simulink model "OuterController"  (R2016b)
settings: Solver=FixedStepAuto  StartTime=0.0  StopTime=t  FixedStep=0.05  RelTol=1e-3
model workspace (MAT data in the model file):
  index = Simulink.Signal
  index.DataType = 'double'
  index.Dimensions = 1
  index.DimensionsMode = 'Fixed'
  index.Complexity = 'real'
  index.SampleTime = -1
  index.SamplingMode = 'auto'
  index.InitialValue = '1'
values from neighbouring files (symbols this model uses):
  AcceptRadius = 1    [Parameters.m]
  wps = [1 0 ... (first row only)    [Parameters.m]
  xbdot = 0.5    [PlannerResults.m]
settings Model: Creator=USUARIO  LastModifiedBy=USUARIO
settings DataIOCC: Refine=100

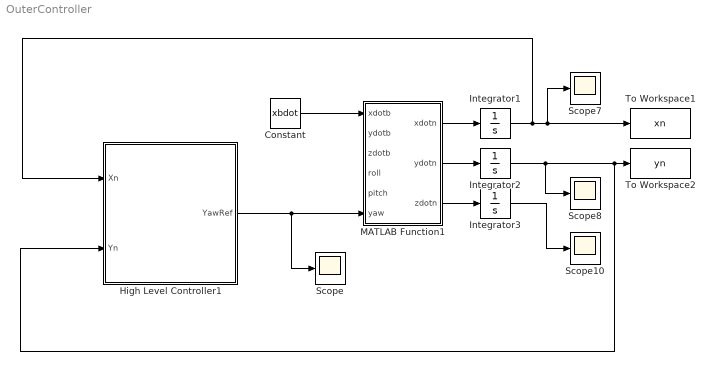
== system OuterController ==
  Constant : Constant  Value=xbdot
  High Level Controller1 : Subsystem
  Integrator1 : Integrator
  Integrator2 : Integrator
  Integrator3 : Integrator
  MATLAB Function1 : MATLAB Function  TreatAsAtomicUnit=on
  Scope{,7..8,10} (4 alike) : Scope
  To Workspace1 : ToWorkspace  VariableName=xn  SaveFormat=Timeseries  SampleTime=-1
  To Workspace2 : ToWorkspace  VariableName=yn  SaveFormat=Timeseries  SampleTime=-1
  wires:
  MATLAB Function1/3(zdotn) -> Integrator3/1
  MATLAB Function1/1(xdotn) -> Integrator1/1
  MATLAB Function1/2(ydotn) -> Integrator2/1
  Integrator3/1 -> Scope10/1
  Integrator1/1 -> High Level Controller1/1(Xn), To Workspace1/1, Scope7/1
  Integrator2/1 -> High Level Controller1/2(Yn), To Workspace2/1, Scope8/1
  High Level Controller1/1(YawRef) -> Scope/1, MATLAB Function1/6(yaw)
  Constant/1 -> MATLAB Function1/1(xdotb)

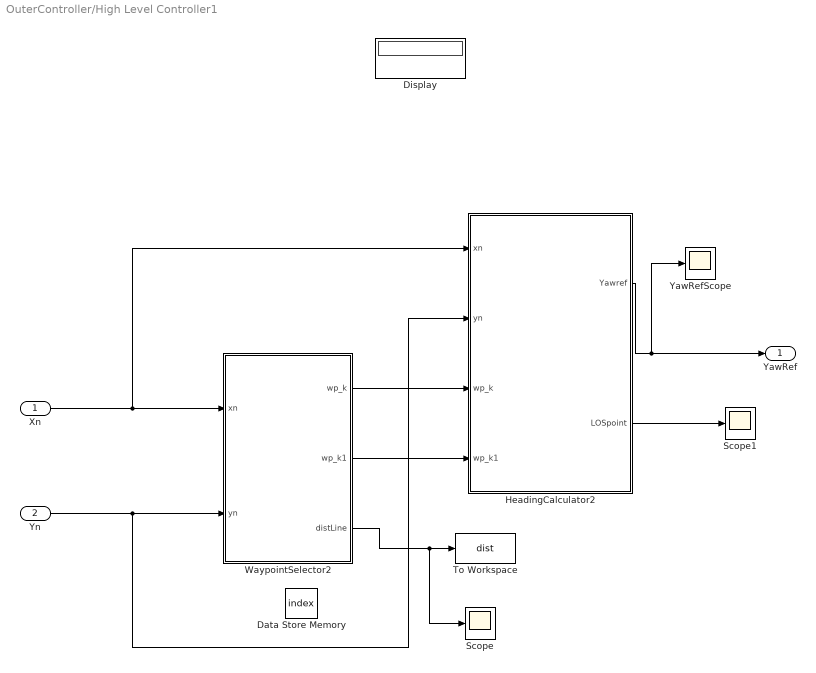
== system OuterController/High Level Controller1 ==
  Xn : Inport  OutDataTypeStr=double  PortDimensions=1
  Yn : Inport  Port=2  OutDataTypeStr=double  PortDimensions=1
  Data Store Memory : DataStoreMemory  DataStoreName=index  ReadBeforeWriteMsg=warning  WriteAfterWriteMsg=warning  WriteAfterReadMsg=warning  InitialValue=1  ShowAdditionalParam=off  OutDataTypeStr=double  Dimensions=1
  Display : Display
  HeadingCalculator2 : MATLAB Function  TreatAsAtomicUnit=on
  Scope : Scope
  Scope1 : Scope
  To Workspace : ToWorkspace  VariableName=dist  SaveFormat=Timeseries  SampleTime=-1
  WaypointSelector2 : MATLAB Function  TreatAsAtomicUnit=on
  YawRefScope : Scope
  YawRef : Outport
  wires:
  Xn/1 -> WaypointSelector2/1(xn), HeadingCalculator2/1(xn)
  Yn/1 -> WaypointSelector2/2(yn), HeadingCalculator2/2(yn)
  HeadingCalculator2/1(Yawref) -> YawRef/1, YawRefScope/1
  WaypointSelector2/1(wp_k) -> HeadingCalculator2/3(wp_k)
  WaypointSelector2/2(wp_k1) -> HeadingCalculator2/4(wp_k1)
  WaypointSelector2/3(distLine) -> Scope/1, To Workspace/1
  HeadingCalculator2/2(LOSpoint) -> Scope1/1

== matlab function OuterController/MATLAB Function1 ==
  data: xdotb input; xdotn output; ydotb input; zdotb input; roll input; pitch input; yaw input; ydotn output; zdotn output
function [xdotn,ydotn,zdotn] = fcn(xdotb,ydotb,zdotb,roll,pitch,yaw)
R=[cos(pitch)*cos(yaw) sin(roll)*sin(pitch)*cos(yaw)-cos(roll)*sin(yaw) ...
                          cos(roll)*sin(pitch)*cos(yaw)+sin(roll)*sin(yaw);
   cos(pitch)*sin(yaw) sin(roll)*sin(pitch)*sin(yaw)+cos(roll)*cos(yaw) ...
                          cos(roll)*sin(pitch)*sin(yaw)-sin(roll)*cos(yaw);
   -sin(pitch) sin(roll)*cos(pitch) cos(roll)*cos(pitch)];

n=R*[xdotb;ydotb;zdotb];

xdotn=n(1);
ydotn=n(2);
zdotn=n(3);
end

== matlab function OuterController/High Level Controller1/HeadingCalculator2 ==
  data: xn input; Yawref output; yn input; wp_k input; wp_k1 input; r parameter; LOSpoint output
function [Yawref, LOSpoint] = HeadingCalculator(xn,yn,wp_k,wp_k1,r)

vessel_pos=[xn,yn];
LOSpoint=FindLOSpoint(wp_k,wp_k1,vessel_pos,r);

Yawref=atan2(LOSpoint(2)-yn,LOSpoint(1)-xn);

== matlab function OuterController/High Level Controller1/WaypointSelector2 ==
  data: xn input; wp_k output; yn input; wp_k1 output; AcceptRadius parameter; wps parameter; index data_store_memory; distLine output
function [wp_k,wp_k1,distLine] = WaypointSelector(xn,yn,AcceptRadius, wps)

global index;

wp_k=wps(index,:);
wp_k1=wps(index+1,:);

[dist,distLine]=FindDistWP(wp_k,wp_k1,[xn,yn]);
if (dist<AcceptRadius) && (size(wps,1)>(index+1))
    index=index+1;
    wp_k=wps(index,:);
    wp_k1=wps(index+1,:);
elseif (size(wps,1)==(index+1))
    xdotref=0; 
end
end
